simulink model "GTC50_DIS"  (R2014b)
settings: Solver=ode3  StartTime=0.0  StopTime=51.6  FixedStep=0.001  RelTol=1e-3
settings Model: Creator=zhoujie  LastModifiedBy=zhoujie

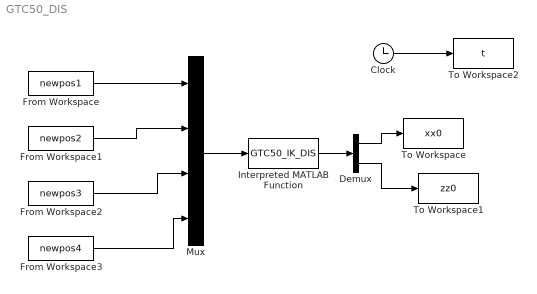
== system GTC50_DIS ==
  Clock : Clock
  Demux : Demux  Outputs=2
  From Workspace : FromWorkspace  VariableName=newpos1  SampleTime=0
  From Workspace1 : FromWorkspace  VariableName=newpos2  SampleTime=0
  From Workspace2 : FromWorkspace  VariableName=newpos3  SampleTime=0
  From Workspace3 : FromWorkspace  VariableName=newpos4  SampleTime=0
  Interpreted MATLAB Function : MATLABFcn  MATLABFcn=GTC50_IK_DIS  OutputDimensions=2
  Mux : Mux
  To Workspace : ToWorkspace  VariableName=xx0  SaveFormat=Timeseries  SampleTime=-1
  To Workspace1 : ToWorkspace  VariableName=zz0  SaveFormat=Timeseries  SampleTime=-1
  To Workspace2 : ToWorkspace  VariableName=t  SaveFormat=Timeseries  SampleTime=-1
  wires:
  From Workspace/1 -> Mux/1
  From Workspace1/1 -> Mux/2
  From Workspace2/1 -> Mux/3
  From Workspace3/1 -> Mux/4
  Mux/1 -> Interpreted MATLAB Function/1
  Interpreted MATLAB Function/1 -> Demux/1
  Demux/1 -> To Workspace/1
  Demux/2 -> To Workspace1/1
  Clock/1 -> To Workspace2/1
